simulink model "Dist_Models_Integrator"  (R2025b)
settings: Solver=VariableStepAuto  StartTime=0.0  StopTime=10.0  RelTol=1e-3
values from neighbouring files (symbols this model uses):
  constantsASTRA = 1.275    [Model_Vars.sldd]
  dt_SIM = 1/500    (= 0.002)    [LoadTOADSim.m]
  r = f ./ f_n    [VRECalc.m]
  x0 = [1; zeros(12,1); constants6DoF.OxMass; constants6DoF.FuMass]    [LoadTOADSim.m]    (also in Model_Vars.sldd = 1.0 0.0 0.0 0.0 0.0 0.0 0.0 0.0 0.0 0.0 0.0 0.0 0.0 20.78 19)
undefined symbols (not defined in the file or in its folder): DiscIntNeverNeededParam, F, Light, MIL
libraries: aerolibwind2 x1
settings Model: Creator=andrew  LastModifiedBy=andrew

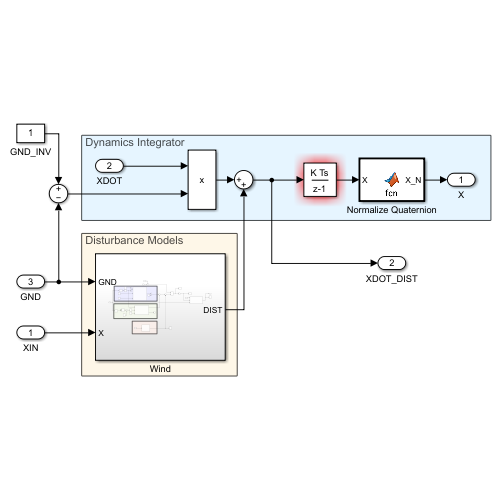
[thumbnail: Simulink's stored preview of the top-level diagram]
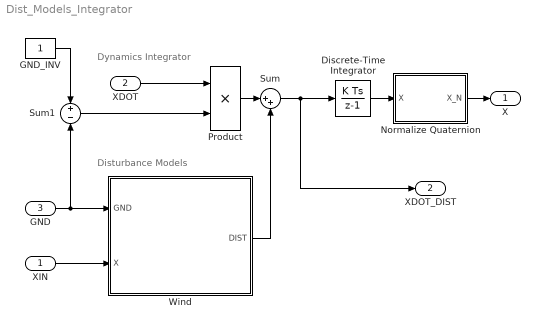
== system Dist_Models_Integrator ==
  note: Dynamics Integrator
  note: Disturbance Models
  XIN : Inport
  XDOT : Inport  Port=2
  GND : Inport  Port=3
  Discrete-Time Integrator : DiscreteIntegrator  InitialCondition=x0  SampleTime=-1  ICPrevOutput=DiscIntNeverNeededParam  ICPrevScaledInput=DiscIntNeverNeededParam
  GND_INV : Constant
  Normalize Quaternion : MATLAB Function  TreatAsAtomicUnit=on
  Product : Product
  Sum : Sum  Inputs=|++
  Sum1 : Sum  Inputs=+|-
  Wind : Subsystem
  X : Outport
  XDOT_DIST : Outport  Port=2
  wires:
  XIN/1 -> Wind/2(X)
  Sum/1 -> Discrete-Time Integrator/1, XDOT_DIST/1
  GND/1 -> Wind/1(GND), Sum1/2
  GND_INV/1 -> Sum1/1
  Sum1/1 -> Product/2
  Normalize Quaternion/1(X_N) -> X/1
  Product/1 -> Sum/1
  XDOT/1 -> Product/1
  Discrete-Time Integrator/1 -> Normalize Quaternion/1(X)
  Wind/1(DIST) -> Sum/2

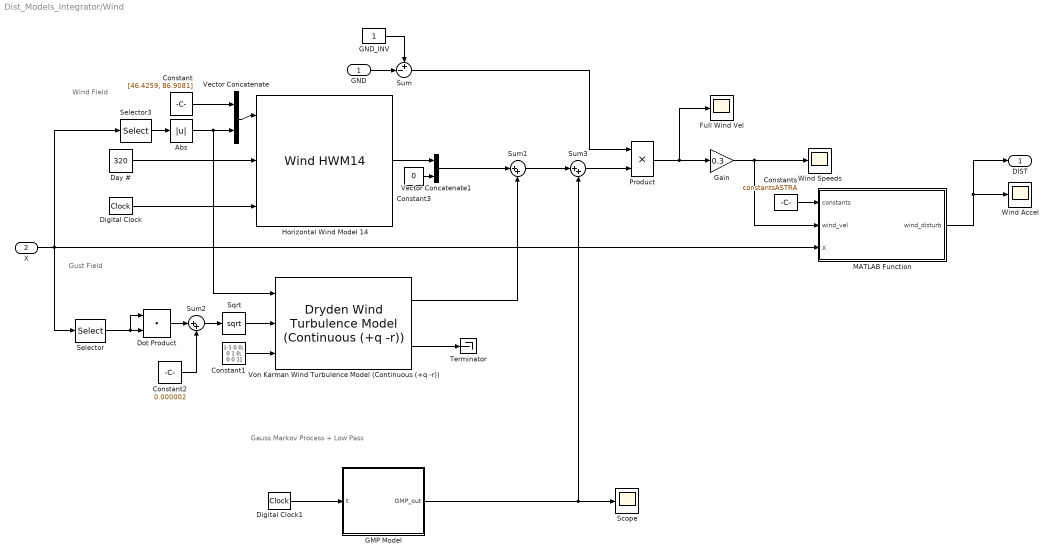
== system Dist_Models_Integrator/Wind ==
  note: Gauss Markov Process + Low Pass
  note: Gust Field
  note: Wind Field
  GND : Inport
  X : Inport  Port=2
  Abs : Abs  SaturateOnIntegerOverflow=off
  Constant : Constant  Value=[46.4259, 86.9081]
  Constant1 : Constant  Value=[-1 0 0; 0 1 0; 0 0 1]
  Constant2 : Constant  Value=0.000002
  Constant3 : Constant  Value=0
  Constants : Constant  Value=constantsASTRA  OutDataTypeStr=Bus: slBus1
  Day # : Constant  Value=320
  Digital Clock : DigitalClock  SampleTime=dt_SIM
  Digital Clock1 : DigitalClock  SampleTime=dt_SIM
  Dot Product : DotProduct  OutDataTypeStr=Inherit: Inherit via internal rule
  Full Wind Vel : Scope
      settings: ActiveDisplayYMinimum=-5.9330847029288414  ActiveDisplayYMaximum=4.4700897462030218  DataLoggingVariableName=ScopeData13
  GMP Model : MATLAB Function  TreatAsAtomicUnit=on
  GND_INV : Constant
  Gain : Gain  Gain=0.3
  Horizontal Wind Model 14 : WindHWM14
  MATLAB Function : MATLAB Function  TreatAsAtomicUnit=on
  Product : Product
  Scope : Scope
      settings: ActiveDisplayYMinimum=-2.8676060433464485  ActiveDisplayYMaximum=2.8612107779538238  DataLoggingVariableName=ScopeData14
  Selector : Selector  InputPortWidth=16  IndexOptions=Index vector (dialog)  Indices=[8:10]  OutputSizes=1
  Selector3 : Selector  InputPortWidth=16  IndexOptions=Index vector (dialog)  Indices=7  OutputSizes=1
  Sqrt : Sqrt
  Sum : Sum  Inputs=+-|
  Sum1 : Sum  Inputs=|++
  Sum2 : Sum  Inputs=|++
  Sum3 : Sum  Inputs=|++
  Terminator : Terminator
  Vector Concatenate : Concatenate
  Vector Concatenate1 : Concatenate
  Von Karman Wind Turbulence Model (Continuous (+q -r)) : aerolibwind2/Dryden Wind Turbulence Model  (Continuous (+q -r))  units=Metric (MKS)  spec=MIL-F-8785C  model=Continuous Von Karman (+q -r)  W20=15  Wdeg=0  TurbProb=10^-2 - Light  L_high=762  Wingspan=10  ts=0.1  Seed=[23341 23342 23343 23344]  T_on=on
      settings: LibrarySourceBlock=|
      | aerolibwind2/Von Karman Wind Turbulence Model
      | (Continuous (+q -r))
  Wind Accel : Scope
      settings: ActiveDisplayYMinimum=-0.93847040858698449  ActiveDisplayYMaximum=0.85102417935944119  DataLoggingVariableName=ScopeData5
  Wind Speeds : Scope
      settings: ActiveDisplayYMinimum=-6.0032131159962416  ActiveDisplayYMaximum=4.44789373969359  DataLoggingVariableName=ScopeData5
  DIST : Outport
  wires:
  Digital Clock/1 -> Horizontal Wind Model 14/3
  Day #/1 -> Horizontal Wind Model 14/2
  MATLAB Function/1(wind_disturb) -> DIST/1, Wind Accel/1
  Vector Concatenate/1 -> Horizontal Wind Model 14/1
  Selector3/1 -> Abs/1
  Constant/1 -> Vector Concatenate/1
  GND/1 -> Sum/2
  Sum/1 -> Product/1
  GND_INV/1 -> Sum/1
  Horizontal Wind Model 14/1 -> Vector Concatenate1/1
  Constants/1 -> MATLAB Function/1(constants)
  Selector/1 -> Dot Product/1, Dot Product/2
  Sqrt/1 -> Von Karman Wind Turbulence Model (Continuous (+q -r))/2
  Von Karman Wind Turbulence Model (Continuous (+q -r))/1 -> Sum1/2
  Constant1/1 -> Von Karman Wind Turbulence Model (Continuous (+q -r))/3
  Sum2/1 -> Sqrt/1
  Dot Product/1 -> Sum2/1
  Constant2/1 -> Sum2/2
  X/1 -> Selector3/1, MATLAB Function/3(X), Selector/1
  Abs/1 -> Vector Concatenate/2, Von Karman Wind Turbulence Model (Continuous (+q -r))/1
  Product/1 -> Full Wind Vel/1, Gain/1
  Vector Concatenate1/1 -> Sum1/1
  Constant3/1 -> Vector Concatenate1/2
  Von Karman Wind Turbulence Model (Continuous (+q -r))/2 -> Terminator/1
  Gain/1 -> Wind Speeds/1, MATLAB Function/2(wind_vel)
  Sum3/1 -> Product/2
  Sum1/1 -> Sum3/1
  GMP Model/1(GMP_out) -> Scope/1, Sum3/2
  Digital Clock1/1 -> GMP Model/1(t)

== matlab function Dist_Models_Integrator/Normalize Quaternion ==
  data: X input; X_N output
function X_N = fcn(X)
X_N = [X(1:4) / norm(X(1:4)); X(5:end)];

== matlab function Dist_Models_Integrator/Wind/GMP Model ==
  data: t input; GMP_out output
function GMP_out = GMP(t)

persistent errorval lastTime EMA
if isempty(errorval)
    errorval = 0;
    EMA = 0;
    lastTime = 0;  % Update last timestamp
end

dT = t - lastTime;

% First order Gauss Markov Process for additional disturbance
decay = 10;
beta = exp(-dT / decay);
covar = 1;
errorval = beta * errorval + sqrt(1 - beta^2) * covar * randn;

% EMA Step to kill High Freq. Noise
EMA = ExpMovingAvg(errorval, EMA, 0.05);
GMP_out = EMA * ones(3,1);
lastTime = t;

== matlab function Dist_Models_Integrator/Wind/MATLAB Function ==
  data: constants input; wind_vel input; X input; wind_disturb output
function wind_disturb = wind_sim(constants, wind_vel, X)

wind_disturb = wind(constants, wind_vel, X);
